simulink model "compare_pidsAAA"  (R2020b)
settings: Solver=VariableStepAuto  StartTime=0.0  StopTime=120  RelTol=1e-3
values from neighbouring files (symbols this model uses):
  kp_cc_strejc = (1.35 / alpha_cc_strejc )*(1 + ((0.18 * tau_cc_strejc)/ (1 - tau_cc_strejc)))    [lab1.m]
  kp_cc_tan = (1.35 / alpha_cc_tan )*(1 + ((0.18 * tau_cc_tan)/ (1 - tau_cc_tan)))    [lab1.m]
  kp_zn1 = 1.2 / a_zn1    [lab1.m]
  td_cc_strejc = ((0.37 - 0.37* tau_cc_strejc)/(1 - 0.81 * tau_cc_strejc)) * l_cc_strejc    [lab1.m]
  td_cc_tan = ((0.37 - 0.37* tau_cc_tan)/(1 - 0.81 * tau_cc_tan)) * l_cc_tan    [lab1.m]
  td_zn1 = l_zn1 / 2    [lab1.m]
  ti_cc_strejc = ((2.50 - 2.0 * tau_cc_strejc)/(1 - 0.39 * tau_cc_strejc)) * l_cc_strejc    [lab1.m]
  ti_cc_tan = ((2.50 - 2.0 * tau_cc_tan)/(1 - 0.39 * tau_cc_tan)) * l_cc_tan    [lab1.m]
  ti_zn1 = 2 * l_zn1    [lab1.m]
undefined symbols (not defined in the file or in its folder): kp_chr_lo_0, kp_chr_lo_20, kp_chr_re_0, kp_chr_re_20, plant_1, td_chr_lo_0, td_chr_lo_20, td_chr_re_0, td_chr_re_20, ti_chr_lo_0, ti_chr_lo_20, ti_chr_re_0, ti_chr_re_20
settings Model: Creator=rafael  LastModifiedBy=rafael

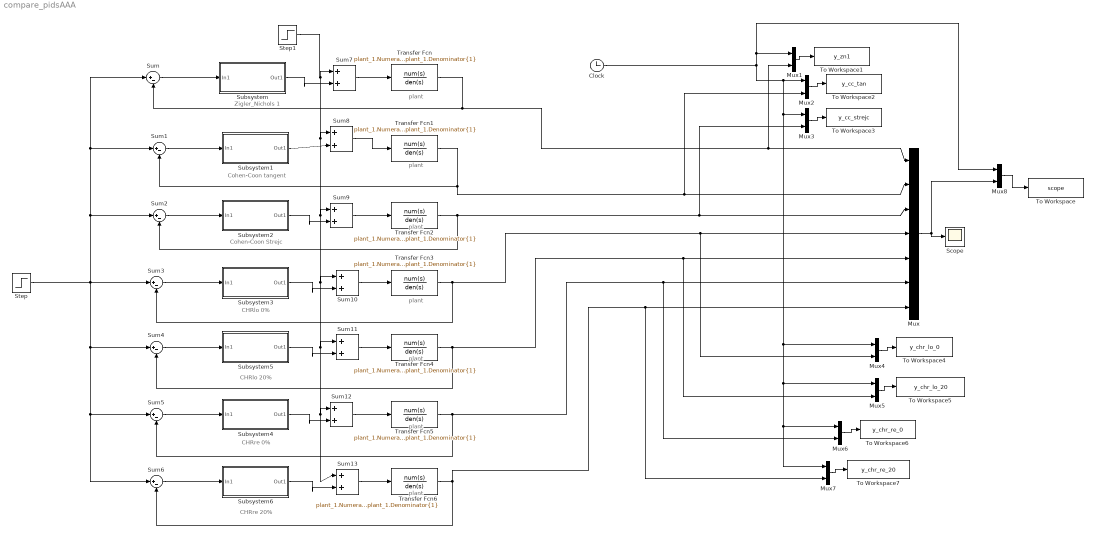
== system compare_pidsAAA ==
  note: plant
  note: Zigler_Nichols 1
  note: Cohen-Coon tangent
  note: Cohen-Coon Strejc
  note: CHRlo 0%
  note: CHRlo 20%
  note: CHRre 0%
  note: CHRre 20%
  note: plant
  note: plant
  note: plant
  note: plant
  note: plant
  note: plant
  Clock : Clock
  Mux : Mux  Inputs=7
  Mux{1..8} (8 alike) : Mux  Inputs=2
  Scope : Scope
  Step : Step  Time=0  SampleTime=0
  Step1 : Step  Time=40  After=-0.5  SampleTime=0
  Subsystem : Subsystem  mask{kp=kp_zn1, ti=ti_zn1, td=td_zn1}
      mask prompts: kp "Proportional gain (kp)"; ti "Integral time (ti)"; td "Derrivative_time (td)"
      mask help: u(s)=kp*(1 + (1/ti)/s + td*s)
      mask Help: /*No help for now*/
      mask Display: disp(' standardPID '), port_label('input',1,'e'), port_label('output',1,'u')
  Subsystem1 : Subsystem  mask{kp=kp_cc_tan, ti=ti_cc_tan, td=td_cc_tan}
      mask prompts: kp "Proportional gain (kp)"; ti "Integral time (ti)"; td "Derrivative_time (td)"
      mask help: u(s)=kp*(1 + (1/ti)/s + td*s)
      mask Help: /*No help for now*/
      mask Display: disp(' standardPID '), port_label('input',1,'e'), port_label('output',1,'u')
  Subsystem2 : Subsystem  mask{kp=kp_cc_strejc, ti=ti_cc_strejc, td=td_cc_strejc}
      mask prompts: kp "Proportional gain (kp)"; ti "Integral time (ti)"; td "Derrivative_time (td)"
      mask help: u(s)=kp*(1 + (1/ti)/s + td*s)
      mask Help: /*No help for now*/
      mask Display: disp(' standardPID '), port_label('input',1,'e'), port_label('output',1,'u')
  Subsystem3 : Subsystem  mask{kp=kp_chr_lo_0, ti=ti_chr_lo_0, td=td_chr_lo_0}
      mask prompts: kp "Proportional gain (kp)"; ti "Integral time (ti)"; td "Derrivative_time (td)"
      mask help: u(s)=kp*(1 + (1/ti)/s + td*s)
      mask Help: /*No help for now*/
      mask Display: disp(' standardPID '), port_label('input',1,'e'), port_label('output',1,'u')
  Subsystem4 : Subsystem  mask{kp=kp_chr_re_0, ti=ti_chr_re_0, td=td_chr_re_0}
      mask prompts: kp "Proportional gain (kp)"; ti "Integral time (ti)"; td "Derrivative_time (td)"
      mask help: u(s)=kp*(1 + (1/ti)/s + td*s)
      mask Help: /*No help for now*/
      mask Display: disp(' standardPID '), port_label('input',1,'e'), port_label('output',1,'u')
  Subsystem5 : Subsystem  mask{kp=kp_chr_lo_20, ti=ti_chr_lo_20, td=td_chr_lo_20}
      mask prompts: kp "Proportional gain (kp)"; ti "Integral time (ti)"; td "Derrivative_time (td)"
      mask help: u(s)=kp*(1 + (1/ti)/s + td*s)
      mask Help: /*No help for now*/
      mask Display: disp(' standardPID '), port_label('input',1,'e'), port_label('output',1,'u')
  Subsystem6 : Subsystem  mask{kp=kp_chr_re_20, ti=ti_chr_re_20, td=td_chr_re_20}
      mask prompts: kp "Proportional gain (kp)"; ti "Integral time (ti)"; td "Derrivative_time (td)"
      mask help: u(s)=kp*(1 + (1/ti)/s + td*s)
      mask Help: /*No help for now*/
      mask Display: disp(' standardPID '), port_label('input',1,'e'), port_label('output',1,'u')
  Sum{,1..6} (7 alike) : Sum  Inputs=|+-
  Sum{7..13} (7 alike) : Sum  Inputs=|++
  To Workspace : ToWorkspace  VariableName=scope  SaveFormat=Timeseries  SampleTime=-1
  To Workspace1 : ToWorkspace  VariableName=y_zn1  SampleTime=-1
      settings: Save2DSignal=2-D array (concatenate along first dimension)
  To Workspace2 : ToWorkspace  VariableName=y_cc_tan  SampleTime=-1
      settings: Save2DSignal=2-D array (concatenate along first dimension)
  To Workspace3 : ToWorkspace  VariableName=y_cc_strejc  SampleTime=-1
      settings: Save2DSignal=2-D array (concatenate along first dimension)
  To Workspace4 : ToWorkspace  VariableName=y_chr_lo_0  SampleTime=-1
      settings: Save2DSignal=2-D array (concatenate along first dimension)
  To Workspace5 : ToWorkspace  VariableName=y_chr_lo_20  SampleTime=-1
      settings: Save2DSignal=2-D array (concatenate along first dimension)
  To Workspace6 : ToWorkspace  VariableName=y_chr_re_0  SampleTime=-1
      settings: Save2DSignal=2-D array (concatenate along first dimension)
  To Workspace7 : ToWorkspace  VariableName=y_chr_re_20  SampleTime=-1
      settings: Save2DSignal=2-D array (concatenate along first dimension)
  Transfer Fcn{,1..6} (7 alike) : TransferFcn  Numerator=plant_1.Numerator{1}  Denominator=plant_1.Denominator{1}
  wires:
  Sum/1 -> Subsystem/1(In1)
  Mux/1 -> Scope/1, Mux8/2
  Sum1/1 -> Subsystem1/1(In1)
  Transfer Fcn1/1 -> Sum1/2, Mux2/2, Mux/2
  Sum2/1 -> Subsystem2/1(In1)
  Transfer Fcn2/1 -> Sum2/2, Mux3/2, Mux/3
  Sum3/1 -> Subsystem3/1(In1)
  Sum4/1 -> Subsystem5/1(In1)
  Transfer Fcn4/1 -> Mux5/2, Mux/5, Sum4/2
  Sum5/1 -> Subsystem4/1(In1)
  Transfer Fcn5/1 -> Mux6/2, Mux/6, Sum5/2
  Sum6/1 -> Subsystem6/1(In1)
  Transfer Fcn6/1 -> Mux/7, Mux7/2, Sum6/2
  Step/1 -> Sum6/1, Sum5/1, Sum4/1, Sum/1, Sum1/1, Sum2/1, Sum3/1
  Mux2/1 -> To Workspace2/1
  Mux1/1 -> To Workspace1/1
  Mux3/1 -> To Workspace3/1
  Transfer Fcn3/1 -> Mux4/2, Mux/4, Sum3/2
  Mux4/1 -> To Workspace4/1
  Clock/1 -> Mux1/1, Mux8/1, Mux4/1, Mux5/1, Mux6/1, Mux7/1, Mux3/1, Mux2/1
  Mux5/1 -> To Workspace5/1
  Mux6/1 -> To Workspace6/1
  Mux7/1 -> To Workspace7/1
  Mux8/1 -> To Workspace/1
  Step1/1 -> Sum13/1, Sum12/1, Sum11/1, Sum10/1, Sum9/1, Sum8/1, Sum7/1
  Subsystem/1(Out1) -> Sum7/2
  Sum7/1 -> Transfer Fcn/1
  Subsystem1/1(Out1) -> Sum8/2
  Sum8/1 -> Transfer Fcn1/1
  Sum9/1 -> Transfer Fcn2/1
  Subsystem2/1(Out1) -> Sum9/2
  Sum13/1 -> Transfer Fcn6/1
  Subsystem6/1(Out1) -> Sum13/2
  Subsystem4/1(Out1) -> Sum12/2
  Subsystem3/1(Out1) -> Sum10/2
  Subsystem5/1(Out1) -> Sum11/2
  Sum10/1 -> Transfer Fcn3/1
  Sum11/1 -> Transfer Fcn4/1
  Sum12/1 -> Transfer Fcn5/1
  Transfer Fcn/1 -> Sum/2, Mux1/2, Mux/1

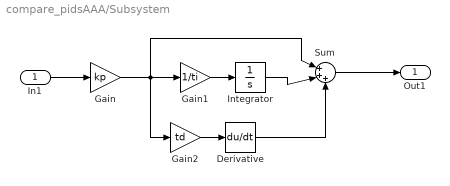
== system compare_pidsAAA/Subsystem ==
  In1 : Inport
  Derivative : Derivative
  Gain : Gain  Gain=kp
  Gain1 : Gain  Gain=1/ti
  Gain2 : Gain  Gain=td
  Integrator : Integrator
  Sum : Sum  Inputs=|+++
  Out1 : Outport
  wires:
  Sum/1 -> Out1/1
  In1/1 -> Gain/1
  Derivative/1 -> Sum/3
  Gain/1 -> Gain2/1, Gain1/1, Sum/1
  Gain2/1 -> Derivative/1
  Integrator/1 -> Sum/2
  Gain1/1 -> Integrator/1

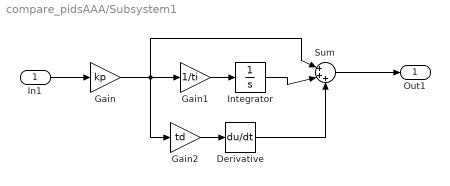
== system compare_pidsAAA/Subsystem1 ==
  In1 : Inport
  Derivative : Derivative
  Gain : Gain  Gain=kp
  Gain1 : Gain  Gain=1/ti
  Gain2 : Gain  Gain=td
  Integrator : Integrator
  Sum : Sum  Inputs=|+++
  Out1 : Outport
  wires:
  Sum/1 -> Out1/1
  In1/1 -> Gain/1
  Derivative/1 -> Sum/3
  Gain/1 -> Gain2/1, Gain1/1, Sum/1
  Gain2/1 -> Derivative/1
  Integrator/1 -> Sum/2
  Gain1/1 -> Integrator/1

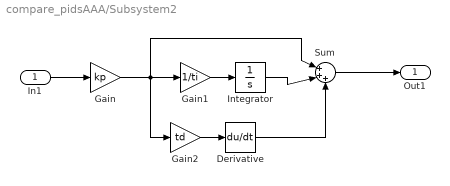
== system compare_pidsAAA/Subsystem2 ==
  In1 : Inport
  Derivative : Derivative
  Gain : Gain  Gain=kp
  Gain1 : Gain  Gain=1/ti
  Gain2 : Gain  Gain=td
  Integrator : Integrator
  Sum : Sum  Inputs=|+++
  Out1 : Outport
  wires:
  Sum/1 -> Out1/1
  In1/1 -> Gain/1
  Derivative/1 -> Sum/3
  Gain/1 -> Gain2/1, Gain1/1, Sum/1
  Gain2/1 -> Derivative/1
  Integrator/1 -> Sum/2
  Gain1/1 -> Integrator/1

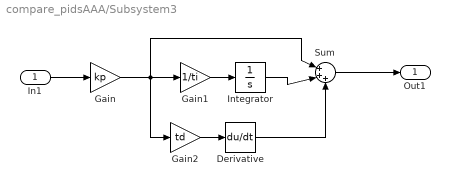
== system compare_pidsAAA/Subsystem3 ==
  In1 : Inport
  Derivative : Derivative
  Gain : Gain  Gain=kp
  Gain1 : Gain  Gain=1/ti
  Gain2 : Gain  Gain=td
  Integrator : Integrator
  Sum : Sum  Inputs=|+++
  Out1 : Outport
  wires:
  Sum/1 -> Out1/1
  In1/1 -> Gain/1
  Derivative/1 -> Sum/3
  Gain/1 -> Gain2/1, Gain1/1, Sum/1
  Gain2/1 -> Derivative/1
  Integrator/1 -> Sum/2
  Gain1/1 -> Integrator/1

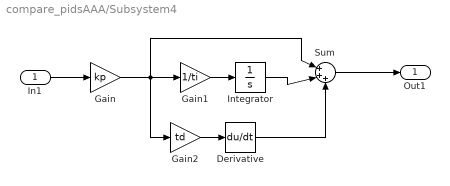
== system compare_pidsAAA/Subsystem4 ==
  In1 : Inport
  Derivative : Derivative
  Gain : Gain  Gain=kp
  Gain1 : Gain  Gain=1/ti
  Gain2 : Gain  Gain=td
  Integrator : Integrator
  Sum : Sum  Inputs=|+++
  Out1 : Outport
  wires:
  Sum/1 -> Out1/1
  In1/1 -> Gain/1
  Derivative/1 -> Sum/3
  Gain/1 -> Gain2/1, Gain1/1, Sum/1
  Gain2/1 -> Derivative/1
  Integrator/1 -> Sum/2
  Gain1/1 -> Integrator/1

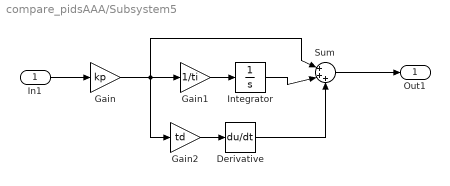
== system compare_pidsAAA/Subsystem5 ==
  In1 : Inport
  Derivative : Derivative
  Gain : Gain  Gain=kp
  Gain1 : Gain  Gain=1/ti
  Gain2 : Gain  Gain=td
  Integrator : Integrator
  Sum : Sum  Inputs=|+++
  Out1 : Outport
  wires:
  Sum/1 -> Out1/1
  In1/1 -> Gain/1
  Derivative/1 -> Sum/3
  Gain/1 -> Gain2/1, Gain1/1, Sum/1
  Gain2/1 -> Derivative/1
  Integrator/1 -> Sum/2
  Gain1/1 -> Integrator/1

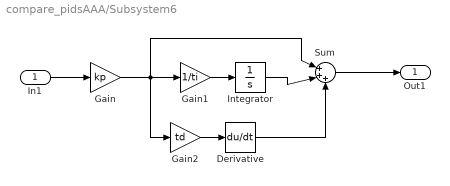
== system compare_pidsAAA/Subsystem6 ==
  In1 : Inport
  Derivative : Derivative
  Gain : Gain  Gain=kp
  Gain1 : Gain  Gain=1/ti
  Gain2 : Gain  Gain=td
  Integrator : Integrator
  Sum : Sum  Inputs=|+++
  Out1 : Outport
  wires:
  Sum/1 -> Out1/1
  In1/1 -> Gain/1
  Derivative/1 -> Sum/3
  Gain/1 -> Gain2/1, Gain1/1, Sum/1
  Gain2/1 -> Derivative/1
  Integrator/1 -> Sum/2
  Gain1/1 -> Integrator/1
